simulink library "dspfdesign"  (Simulink 8.3)
settings: Solver=ode45  SolverMode=SingleTasking  StartTime=0.0  StopTime=10.0  RelTol=1e-3
undefined symbols (not defined in the file or in its folder): dfilt, fdesignblkfcn, gcbh
libraries: dsparch4 x4, dspmlti4 x1
settings Model: FPTRunName=Active  Creator=jschickl  LastModifiedBy=jibrahim  ExtModeAutoUpdateStatusClock=off

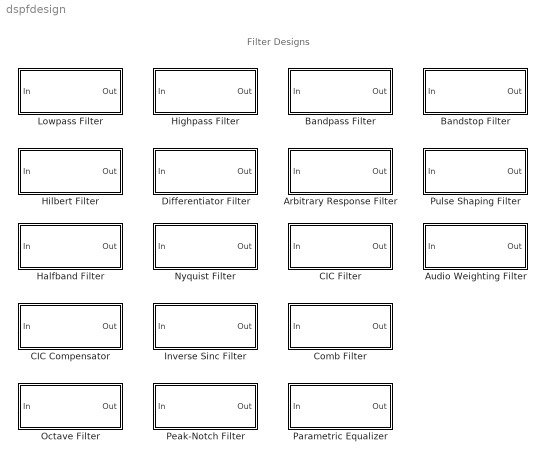
== system dspfdesign ==
  note: Filter Designs
  Arbitrary Response Filter : Subsystem  DialogController=fdesignblkfcn  DialogControllerArgs=DataTag1  InitFcn=fdesignblkfcn(gcbh, {'InitFcn'});  mask(Arbitrary Magnitude Filter){}
      mask help: Design an arbitrary magnitude filter
      settings: CopyFcn=fdesignblkfcn(gcbh, {'CopyFcn'});
      mask Help: helpview(mapfilelocation('dsp'), 'dsparbitrarymagnitudefilter');
      mask Display: disp('Arbitrary Response');
  Audio Weighting Filter : Subsystem  DialogController=fdesignblkfcn  DialogControllerArgs=DataTag3  InitFcn=fdesignblkfcn(gcbh, {'InitFcn'});  mask(Audio Weighting Filter){}
      mask help: Design an audio weighting filter
      settings: CopyFcn=fdesignblkfcn(gcbh, {'CopyFcn'});
      mask Help: helpview(mapfilelocation('dsp'), 'dspaudioweightingfilter');
      mask Display: disp('Audio Weighting')
  Bandpass Filter : Subsystem  DialogController=fdesignblkfcn  DialogControllerArgs=DataTag6  InitFcn=fdesignblkfcn(gcbh, {'InitFcn'});  mask(Bandpass Filter){}
      mask help: Design a bandpass filter
      settings: CopyFcn=fdesignblkfcn(gcbh, {'CopyFcn'});
      mask Help: helpview(mapfilelocation('dsp'), 'dspbandpassfilter');
      mask Display: disp('Bandpass');
  Bandstop Filter : Subsystem  DialogController=fdesignblkfcn  DialogControllerArgs=DataTag8  InitFcn=fdesignblkfcn(gcbh, {'InitFcn'});  mask(Bandstop Filter){}
      mask help: Design a bandstop filter
      settings: CopyFcn=fdesignblkfcn(gcbh, {'CopyFcn'});
      mask Help: helpview(mapfilelocation('dsp'), 'dspbandstopfilter');
      mask Display: disp('Bandstop');
  CIC Compensator : Subsystem  DialogController=fdesignblkfcn  DialogControllerArgs=DataTag10  InitFcn=fdesignblkfcn(gcbh, {'InitFcn'});  mask(CIC Compensator){}
      mask help: Design a CIC compensator
      settings: CopyFcn=fdesignblkfcn(gcbh, {'CopyFcn'});
      mask Help: helpview(mapfilelocation('dsp'), 'dspciccompensator');
      mask Display: disp('CIC Comp.')
  CIC Filter : Subsystem  DialogController=fdesignblkfcn  DialogControllerArgs=DataTag12  InitFcn=fdesignblkfcn(gcbh, {'InitFcn'});  mask(CIC Filter){}
      mask help: Design a CIC filter
      settings: CopyFcn=fdesignblkfcn(gcbh, {'CopyFcn'});
      mask Help: helpview(mapfilelocation('dsp'), 'dspcicfilter');
      mask Display: disp('CIC')
  Comb Filter : Subsystem  DialogController=fdesignblkfcn  DialogControllerArgs=DataTag15  InitFcn=fdesignblkfcn(gcbh, {'InitFcn'});  mask(Comb Filter){}
      mask help: Design a Comb Filter
      settings: CopyFcn=fdesignblkfcn(gcbh, {'CopyFcn'});
      mask Help: helpview(mapfilelocation('dsp'), 'dspcombfilter');
      mask Display: disp('Comb');
  Differentiator Filter : Subsystem  DialogController=fdesignblkfcn  DialogControllerArgs=DataTag17  InitFcn=fdesignblkfcn(gcbh, {'InitFcn'});  mask(Differentiator Filter){}
      mask help: Design a differentiator filter
      settings: CopyFcn=fdesignblkfcn(gcbh, {'CopyFcn'});
      mask Help: helpview(mapfilelocation('dsp'), 'dspdifferentiatorfilter');
      mask Display: disp('Differentiator');
  Halfband Filter : Subsystem  DialogController=fdesignblkfcn  DialogControllerArgs=DataTag19  InitFcn=fdesignblkfcn(gcbh, {'InitFcn'});  mask(Halfband Filter){}
      mask help: Design a halfband filter
      settings: CopyFcn=fdesignblkfcn(gcbh, {'CopyFcn'});
      mask Help: helpview(mapfilelocation('dsp'), 'dsphalfbandfilter');
      mask Display: disp('Halfband');
  Highpass Filter : Subsystem  DialogController=fdesignblkfcn  DialogControllerArgs=DataTag21  InitFcn=fdesignblkfcn(gcbh, {'InitFcn'});  mask(Highpass Filter){}
      mask help: Design a highpass filter
      settings: CopyFcn=fdesignblkfcn(gcbh, {'CopyFcn'});
      mask Help: helpview(mapfilelocation('dsp'), 'dsphighpassfilter');
      mask Display: disp('Highpass')
  Hilbert Filter : Subsystem  DialogController=fdesignblkfcn  DialogControllerArgs=DataTag23  InitFcn=fdesignblkfcn(gcbh, {'InitFcn'});  mask(Hilbert Filter){}
      mask help: Design a Hilbert filter
      settings: CopyFcn=fdesignblkfcn(gcbh, {'CopyFcn'});
      mask Help: helpview(mapfilelocation('dsp'), 'dsphilbertfilter');
      mask Display: disp('Hilbert')
  Inverse Sinc Filter : Subsystem  DialogController=fdesignblkfcn  DialogControllerArgs=DataTag25  InitFcn=fdesignblkfcn(gcbh, {'InitFcn'});  mask(Inverse Sinc Filter){}
      mask help: Design an inverse sinc filter
      settings: CopyFcn=fdesignblkfcn(gcbh, {'CopyFcn'});
      mask Help: helpview(mapfilelocation('dsp'), 'dspinversesincfilter');
      mask Display: disp('Inverse Sinc');
  Lowpass Filter : Subsystem  DialogController=fdesignblkfcn  DialogControllerArgs=DataTag27  InitFcn=fdesignblkfcn(gcbh, {'InitFcn'});  mask(Lowpass Filter){}
      mask help: Design a lowpass filter
      settings: CopyFcn=fdesignblkfcn(gcbh, {'CopyFcn'});
      mask Help: helpview(mapfilelocation('dsp'), 'dsplowpassfilter');
      mask Display: disp('Lowpass')
  Nyquist Filter : Subsystem  DialogController=fdesignblkfcn  DialogControllerArgs=DataTag29  InitFcn=fdesignblkfcn(gcbh, {'InitFcn'});  mask(Nyquist Filter){}
      mask help: Design a Nyquist filter
      settings: CopyFcn=fdesignblkfcn(gcbh, {'CopyFcn'});
      mask Help: helpview(mapfilelocation('dsp'), 'dspnyquistfilter');
      mask Display: disp('Nyquist');
  Octave Filter : Subsystem  DialogController=fdesignblkfcn  DialogControllerArgs=DataTag31  InitFcn=fdesignblkfcn(gcbh, {'InitFcn'});  mask(Octave Filter){}
      mask help: Design an octave filter
      settings: CopyFcn=fdesignblkfcn(gcbh, {'CopyFcn'});
      mask Help: helpview(mapfilelocation('dsp'), 'dspoctavefilter');
      mask Display: disp('Octave');
  Parametric Equalizer : Subsystem  DialogController=fdesignblkfcn  DialogControllerArgs=DataTag34  InitFcn=fdesignblkfcn(gcbh, {'InitFcn'});  mask(Parametric Equalizer){}
      mask help: Design a parametric equalizer
      settings: CopyFcn=fdesignblkfcn(gcbh, {'CopyFcn'});
      mask Help: helpview(mapfilelocation('dsp'), 'dspparametricequalizer');
      mask Display: disp('Param Eq');
  Peak-Notch Filter : Subsystem  DialogController=fdesignblkfcn  DialogControllerArgs=DataTag37  InitFcn=fdesignblkfcn(gcbh, {'InitFcn'});  mask(Peak/Notch Filter){}
      mask help: Design a peak/notch filter
      settings: CopyFcn=fdesignblkfcn(gcbh, {'CopyFcn'});
      mask Help: helpview(mapfilelocation('dsp'), 'dsppeaknotchfilter');
      mask Display: disp('Peak-Notch');
  Pulse Shaping Filter : Subsystem  DialogController=fdesignblkfcn  DialogControllerArgs=DataTag40  InitFcn=fdesignblkfcn(gcbh, {'InitFcn'});  mask(Pulse Shaping Filter){}
      mask help: Design a Pulse Shaping Filter
      settings: CopyFcn=fdesignblkfcn(gcbh, {'CopyFcn'});
      mask Help: helpview(mapfilelocation('dsp'), 'dsppulseshapingfilter');
      mask Display: disp('Pulse Shaping');

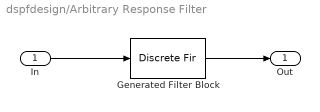
== system dspfdesign/Arbitrary Response Filter ==
  In : Inport
  Generated Filter Block : DiscreteFir  Tag=BlockMethodSubSystem  Coefficients=[-6.0602616490905374e-17 -0.030302449967817502 -2.7240579583698299e-18 -0.042316580413584839 1.9768060143351985e-17 -0.1094403863154082 6.5949666030061724e-17 0.28666822580143747 -9.0831528312516844e-17 0.093783802666672023 0.5 0.093783802666671731 1.4840405705753284e-16 0.28666822580143747 -1.1769252026794985e-16 -0.10944038631540809 3.1431295905226604e-17 -0.042316580413584826 -8.227645756848666e-17 -0.030302449967817453 1.2107664253565005e-16]  InputProcessing=Columns as channels (frame based)
  Out : Outport
  wires:
  In/1 -> Generated Filter Block/1
  Generated Filter Block/1 -> Out/1

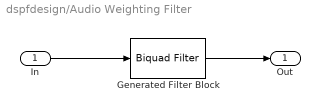
== system dspfdesign/Audio Weighting Filter ==
  In : Inport
  Generated Filter Block : dsparch4/Biquad Filter  Tag=BlockMethodSubSystem  IIRFiltStruct=Direct form II  CoeffSource=Specify via dialog  BiQuadCoeffs=[0.000322318592897719 0.000644637185795438 0.000322318592897719 1 -0.224558458059779 0.0126066252715464;1 -2 1 1 -1.89387049472307 0.895159769094661;1 -2 1 1 -1.99461445599302 0.994621707014084]  a0Flag=Warning  IC=0  ICnum=0  ICden=0  InputProcessing=Columns as channels (frame based)  denAccumFracLength=30  denProdOutputFracLength=30  secondMemoryFracLength=15  roundingMode=Floor  overflowMode=off  ScaleValues=[0.788048167211767;1;1;922.438644632257]  optimizeScaleValues=off  ScaleValueMode=Specify via input port (g)  scaleValueFracLength=14  FilterSource=Specify via dialog  dfiltObjectName=dfilt.df2tsos([1 0.3 0.4],[1 0.1 0.2])
  Out : Outport
  wires:
  Generated Filter Block/1 -> Out/1
  In/1 -> Generated Filter Block/1

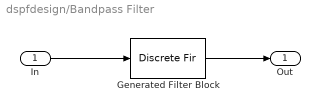
== system dspfdesign/Bandpass Filter ==
  In : Inport
  Generated Filter Block : DiscreteFir  Tag=BlockMethodSubSystem  Coefficients=[-0.0008992291487744296 0.0016414518747943749 0.0031352071842225397 -0.0040707550828814922 -0.0063731852227904111 0.0074874286806090491 0.0098354319566295711 -0.010189316513446216 -0.011302794465874122 0.0096929185841818435 0.0079428653987464216 -0.0031368247881221642 0.0028299878877943137 -0.011508674243001471 -0.022080136219461581 0.034245325424507672 0.048356661648905473 -0.062355369169884239 -0.077503478162593897 0.090687768153125653 0.10353171105844157 -0.11297860084229834 -0.12035866024978455 0.12379360801539134 0.12379360801539134 -0.12035866024978455 -0.11297860084229834 0.10353171105844157 0.090687768153125653 -0.077503478162593897 -0.062355369169884239 0.048356661648905473 0.034245325424507672 -0.022080136219461581 -0.011508674243001471 0.0028299878877943137 -0.0031368247881221642 0.0079428653987464216 0.0096929185841818435 -0.011302794465874122 -0.010189316513446216 0.0098354319566295711 0.0074874286806090491 -0.0063731852227904111 -0.0040707550828814922 0.0031352071842225397 0.0016414518747943749 -0.0008992291487744296]  InputProcessing=Columns as channels (frame based)
  Out : Outport
  wires:
  Generated Filter Block/1 -> Out/1
  In/1 -> Generated Filter Block/1

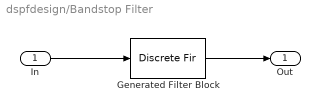
== system dspfdesign/Bandstop Filter ==
  In : Inport
  Generated Filter Block : DiscreteFir  Tag=BlockMethodSubSystem  Coefficients=[-0.00049984690227566171 9.5100318056220678e-05 -0.018778888889125381 0.00020561736622238936 0.0019605411941885044 0.00023848464356614288 0.011427768692370117 0.00024928020776728103 -0.026344143468356181 0.00022323473160311075 0.033802321854574921 0.00024455404571586617 -0.019823660150560137 0.00024377045334422507 -0.019896328302992174 0.00022786848806407702 0.082714162332194516 0.00025656261277749384 -0.15101859373266049 0.00022072984516862497 0.20526035643478094 0.0002476136866061962 0.77489283142488197 0.0002476136866061962 0.20526035643478094 0.00022072984516862497 -0.15101859373266049 0.00025656261277749384 0.082714162332194516 0.00022786848806407702 -0.019896328302992174 0.00024377045334422507 -0.019823660150560137 0.00024455404571586617 0.033802321854574921 0.00022323473160311075 -0.026344143468356181 0.00024928020776728103 0.011427768692370117 0.00023848464356614288 0.0019605411941885044 0.00020561736622238936 -0.018778888889125381 9.5100318056220678e-05 -0.00049984690227566171]  InputProcessing=Columns as channels (frame based)
  Out : Outport
  wires:
  In/1 -> Generated Filter Block/1
  Generated Filter Block/1 -> Out/1

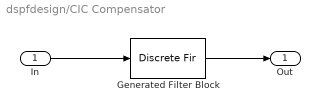
== system dspfdesign/CIC Compensator ==
  In : Inport
  Generated Filter Block : DiscreteFir  Tag=BlockMethodSubSystem  Coefficients=[-0.0050219629876821908 -0.013660028067670223 -0.013296841217015732 0.0011859158588442293 0.011467493725642241 -0.00013417577627168609 -0.013874989743002046 -0.0015600948868864728 0.0180127865455753 0.0042866842548780126 -0.023312910868604299 -0.0087360042158460029 0.030313491605369943 0.015598915258060758 -0.039779435104977612 -0.027013109649543846 0.054210638861692181 0.048428131419013934 -0.08074386512301486 -0.10321504031178634 0.15358183075835236 0.46749760644592786 0.46749760644592786 0.15358183075835236 -0.10321504031178634 -0.08074386512301486 0.048428131419013934 0.054210638861692181 -0.027013109649543846 -0.039779435104977612 0.015598915258060758 0.030313491605369943 -0.0087360042158460029 -0.023312910868604299 0.0042866842548780126 0.0180127865455753 -0.0015600948868864728 -0.013874989743002046 -0.00013417577627168609 0.011467493725642241 0.0011859158588442293 -0.013296841217015732 -0.013660028067670223 -0.0050219629876821908]  InputProcessing=Columns as channels (frame based)
  Out : Outport
  wires:
  In/1 -> Generated Filter Block/1
  Generated Filter Block/1 -> Out/1

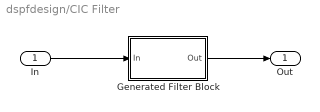
== system dspfdesign/CIC Filter ==
  In : Inport
  Generated Filter Block : Subsystem  Tag=BlockMethodSubSystem
  Out : Outport
  wires:
  Generated Filter Block/1(Out) -> Out/1
  In/1 -> Generated Filter Block/1(In)

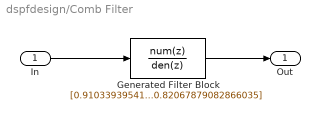
== system dspfdesign/Comb Filter ==
  In : Inport
  Generated Filter Block : DiscreteFilter  Tag=BlockMethodSubSystem  Numerator=[0.91033939541433018 0 0 0 0 0 0 0 0 0 -0.91033939541433018]  Denominator=[1 0 0 0 0 0 0 0 0 0 -0.82067879082866035]  InputProcessing=Columns as channels (frame based)
  Out : Outport
  wires:
  In/1 -> Generated Filter Block/1
  Generated Filter Block/1 -> Out/1

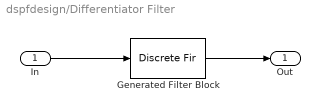
== system dspfdesign/Differentiator Filter ==
  In : Inport
  Generated Filter Block : DiscreteFir  Tag=BlockMethodSubSystem  Coefficients=[-0.0039403783503444709 0.0053805058704480841 -0.0026652365685344249 0.0025070872881500926 -0.0027292449144808066 0.0031396751895010648 -0.0037469771156754452 0.0046041330268851155 -0.0058435320681063689 0.007709493104211795 -0.010689468560152578 0.015879080885195844 -0.026138778807662393 0.051078874208799696 -0.14161732347277556 1.2733839756566323 -1.2733839756566323 0.14161732347277556 -0.051078874208799696 0.026138778807662393 -0.015879080885195844 0.010689468560152578 -0.007709493104211795 0.0058435320681063689 -0.0046041330268851155 0.0037469771156754452 -0.0031396751895010648 0.0027292449144808066 -0.0025070872881500926 0.0026652365685344249 -0.0053805058704480841 0.0039403783503444709]  InputProcessing=Columns as channels (frame based)
  Out : Outport
  wires:
  In/1 -> Generated Filter Block/1
  Generated Filter Block/1 -> Out/1

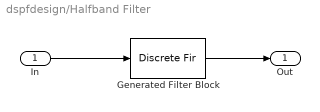
== system dspfdesign/Halfband Filter ==
  In : Inport
  Generated Filter Block : DiscreteFir  Tag=BlockMethodSubSystem  Coefficients=[-8.9481765259157725e-05 0 0.00013477350905337501 0 -0.0002322836857224922 0 0.00037237197523475751 0 -0.00056658311312798111 0 0.00082825383475131466 0 -0.0011725457806439315 0 0.0016168803439530585 0 -0.0021808856576991135 0 0.0028874400591769505 0 -0.0037630129230021257 0 0.0048394806436799498 0 -0.0061564154803690867 0 0.0077647763061666625 0 -0.009733715050901065 0 0.012161878543157797 0 -0.015198123798392082 0 0.019081615239417135 0 -0.024225970822374349 0 0.031415272990123339 0 -0.042336185081318312 0 0.061387315847790502 0 -0.10472460953008161 0 0.31784798756502125 0.5 0.31784798756502125 0 -0.10472460953008161 0 0.061387315847790502 0 -0.042336185081318312 0 0.031415272990123339 0 -0.024225970822374349 0 0.019081615239417135 0 -0.015198123798392082 0 0.012161878543157797 0 -0.009733715050901065 0 0.0077647763061666625 0 -0.0061564154803690867 0 0.0048394806436799498 0 -0.0037630129230021257 0 0.0028874400591769505 0 -0.0021808856576991135 0 0.0016168803439530585 0 -0.0011725457806439315 0 0.00082825383475131466 0 -0.00056658311312798111 0 0.00037237197523475751 0 -0.0002322836857224922 0 0.00013477350905337501 0 -8.9481765259157725e-05]  InputProcessing=Columns as channels (frame based)
  Out : Outport
  wires:
  In/1 -> Generated Filter Block/1
  Generated Filter Block/1 -> Out/1

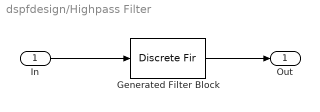
== system dspfdesign/Highpass Filter ==
  In : Inport
  Generated Filter Block : DiscreteFir  Tag=BlockMethodSubSystem  Coefficients=[-0.001713682665110306 0.0083143784480805769 -0.012717355233486931 0.0055609517902503753 0.0073397102425536197 -0.006531049050179258 -0.0076900499697794954 0.0090269831680985079 0.0088388618995090904 -0.012960741353766195 -0.010074958667252783 0.018520174010008873 0.011233354613588929 -0.026375248383613631 -0.012270782185765867 0.038180976692389727 0.013130425918293593 -0.058293359325192265 -0.013768295948648092 0.102813257992074 0.014167876773854067 -0.31720255241603534 0.48569804617051759 -0.31720255241603534 0.014167876773854067 0.102813257992074 -0.013768295948648092 -0.058293359325192265 0.013130425918293593 0.038180976692389727 -0.012270782185765867 -0.026375248383613631 0.011233354613588929 0.018520174010008873 -0.010074958667252783 -0.012960741353766195 0.0088388618995090904 0.0090269831680985079 -0.0076900499697794954 -0.006531049050179258 0.0073397102425536197 0.0055609517902503753 -0.012717355233486931 0.0083143784480805769 -0.001713682665110306]  InputProcessing=Columns as channels (frame based)
  Out : Outport
  wires:
  In/1 -> Generated Filter Block/1
  Generated Filter Block/1 -> Out/1

== system dspfdesign/Hilbert Filter ==
  In : Inport
  Generated Filter Block : DiscreteFir  Tag=BlockMethodSubSystem  Coefficients=[-0.026449858259791379 -0.00578355491829027 -0.016572261903348456 -0.0095390561131982743 -0.022461390535071568 -0.014999256435125952 -0.030323967074738556 -0.023012528163449009 -0.041429315821655127 -0.035762828939278346 -0.05911752381753177 -0.059034685410808696 -0.094459906652176406 -0.11739830204172252 -0.21797718993610349 -0.62869353747279177 0.62869353747279177 0.21797718993610349 0.11739830204172252 0.094459906652176406 0.059034685410808696 0.05911752381753177 0.035762828939278346 0.041429315821655127 0.023012528163449009 0.030323967074738556 0.014999256435125952 0.022461390535071568 0.0095390561131982743 0.016572261903348456 0.00578355491829027 0.026449858259791379]  InputProcessing=Columns as channels (frame based)
  Out : Outport
  wires:
  In/1 -> Generated Filter Block/1
  Generated Filter Block/1 -> Out/1

== system dspfdesign/Inverse Sinc Filter ==
  In : Inport
  Generated Filter Block : DiscreteFir  Tag=BlockMethodSubSystem  Coefficients=[-0.0026843274692852663 -0.002346162151096788 0.0073965993169508026 0.018442797618651186 0.012351106329410911 -0.0067934613704367722 -0.0093225132104399755 0.010137634289690594 0.014452636598032568 -0.01096659610710831 -0.020288876931548214 0.012277085521236011 0.029020142443779536 -0.013203596820367916 -0.042093940662690496 0.013627754834690312 0.064277570694568714 -0.012757715101713234 -0.11270171800644833 0.0051188971746040065 0.32344134739197722 0.50160314889955848 0.32344134739197722 0.0051188971746040065 -0.11270171800644833 -0.012757715101713234 0.064277570694568714 0.013627754834690312 -0.042093940662690496 -0.013203596820367916 0.029020142443779536 0.012277085521236011 -0.020288876931548214 -0.01096659610710831 0.014452636598032568 0.010137634289690594 -0.0093225132104399755 -0.0067934613704367722 0.012351106329410911 0.018442797618651186 0.0073965993169508026 -0.002346162151096788 -0.0026843274692852663]  InputProcessing=Columns as channels (frame based)
  Out : Outport
  wires:
  In/1 -> Generated Filter Block/1
  Generated Filter Block/1 -> Out/1

== system dspfdesign/Lowpass Filter ==
  In : Inport
  Generated Filter Block : DiscreteFir  Tag=BlockMethodSubSystem  Coefficients=[-0.0024228738523269142 -0.002083244982079274 0.0067703446401187091 0.016731945423489058 0.011117076081077608 -0.0062311454141445394 -0.008401617186026911 0.0092567976151380175 0.012982883808855752 -0.010121234703278968 -0.018273518733782485 0.011431962071777957 0.02617588858040763 -0.012489027835322923 -0.037996623145463579 0.013388945199366963 0.058155465814729891 -0.014048043515808939 -0.10272466857882172 0.014462275771238358 0.31716649721769491 0.48538764678732504 0.31716649721769491 0.014462275771238358 -0.10272466857882172 -0.014048043515808939 0.058155465814729891 0.013388945199366963 -0.037996623145463579 -0.012489027835322923 0.02617588858040763 0.011431962071777957 -0.018273518733782485 -0.010121234703278968 0.012982883808855752 0.0092567976151380175 -0.008401617186026911 -0.0062311454141445394 0.011117076081077608 0.016731945423489058 0.0067703446401187091 -0.002083244982079274 -0.0024228738523269142]  InputProcessing=Columns as channels (frame based)
  Out : Outport
  wires:
  Generated Filter Block/1 -> Out/1
  In/1 -> Generated Filter Block/1

== system dspfdesign/Nyquist Filter ==
  In : Inport
  Generated Filter Block : DiscreteFir  Tag=BlockMethodSubSystem  Coefficients=[-1.5162272612995586e-05 0 4.1706564279713027e-05 0 -8.6397453235949307e-05 0 0.00015611233941239259 0 -0.00025915216340561289 0 0.00040534096772710702 0 -0.00060612208112690072 0 0.00087466461351889491 0 -0.0012260032157642615 0 0.0016772472887656247 0 -0.0022479153417375975 0 0.002960480176087802 0 -0.0038412587047380814 0 0.0049218611113159959 0 -0.0062415564318662039 0 0.0078511744671022864 0 -0.0098196745838436145 0 0.012245562776669343 0 -0.015277650505299337 0 0.019155163922055268 0 -0.024291754943524414 0 0.031471599148898237 0 -0.042381607242685339 0 0.061420660829271646 0 -0.10474499179295332 0 0.31785484611193615 0.5 0.31785484611193615 0 -0.10474499179295332 0 0.061420660829271646 0 -0.042381607242685339 0 0.031471599148898237 0 -0.024291754943524414 0 0.019155163922055268 0 -0.015277650505299337 0 0.012245562776669343 0 -0.0098196745838436145 0 0.0078511744671022864 0 -0.0062415564318662039 0 0.0049218611113159959 0 -0.0038412587047380814 0 0.002960480176087802 0 -0.0022479153417375975 0 0.0016772472887656247 0 -0.0012260032157642615 0 0.00087466461351889491 0 -0.00060612208112690072 0 0.00040534096772710702 0 -0.00025915216340561289 0 0.00015611233941239259 0 -8.6397453235949307e-05 0 4.1706564279713027e-05 0 -1.5162272612995586e-05]  InputProcessing=Columns as channels (frame based)
  Out : Outport
  wires:
  Generated Filter Block/1 -> Out/1
  In/1 -> Generated Filter Block/1

== system dspfdesign/Octave Filter ==
  In : Inport
  Generated Filter Block : dsparch4/Biquad Filter  Tag=BlockMethodSubSystem  IIRFiltStruct=Direct form II  CoeffSource=Specify via dialog  BiQuadCoeffs=[0.115971860617354 0 -0.115971860617354 1 -1.95883566965961 0.967994525760731;0.0548911505711939 0 -0.0548911505711939 1 -1.91157093401714 0.942106946582538;2 0 -2 1 -1.89540803000166 0.911775131877275]  a0Flag=Warning  IC=0  ICnum=0  ICden=0  InputProcessing=Columns as channels (frame based)  denAccumFracLength=30  denProdOutputFracLength=30  secondMemoryFracLength=15  roundingMode=Floor  overflowMode=off  ScaleValues=[0.00304051963098346;1;1;2.31504954634773]  optimizeScaleValues=off  ScaleValueMode=Specify via input port (g)  scaleValueFracLength=14  FilterSource=Specify via dialog  dfiltObjectName=dfilt.df2tsos([1 0.3 0.4],[1 0.1 0.2])
  Out : Outport
  wires:
  In/1 -> Generated Filter Block/1
  Generated Filter Block/1 -> Out/1

== system dspfdesign/Parametric Equalizer ==
  In : Inport
  Generated Filter Block : dsparch4/Biquad Filter  Tag=BlockMethodSubSystem  IIRFiltStruct=Direct form II  CoeffSource=Specify via dialog  BiQuadCoeffs=[0.848020960436601 0.659110935021998 0.38962445572443 1 0.55108714605605 0.621190092613526;1.60063898438456 -1.24407144027101 0.735415894414984 1 -0.551087146056049 0.621190092613524]  a0Flag=Warning  IC=0  ICnum=0  ICden=0  InputProcessing=Columns as channels (frame based)  denAccumFracLength=30  denProdOutputFracLength=30  secondMemoryFracLength=15  roundingMode=Floor  overflowMode=off  ScaleValues=[0.35490589484659;1;1]  optimizeScaleValues=off  ScaleValueMode=Specify via input port (g)  scaleValueFracLength=14  FilterSource=Specify via dialog  dfiltObjectName=dfilt.df2tsos([1 0.3 0.4],[1 0.1 0.2])
  Out : Outport
  wires:
  In/1 -> Generated Filter Block/1
  Generated Filter Block/1 -> Out/1

== system dspfdesign/Peak-Notch Filter ==
  In : Inport
  Generated Filter Block : dsparch4/Biquad Filter  Tag=BlockMethodSubSystem  IIRFiltStruct=Direct form II  CoeffSource=Specify via dialog  BiQuadCoeffs=[0.38547134611574 -0.77094269223148 0.38547134611574 1 0.476387796295706 0.738730881654112;0.307522030597872 -4.58243541688184e-09 -0.307522026015436 1 -0.476387796295706 0.73873088165411;0.608203917574429 1.2164078442118 0.608203926637374 1 0 0.509525449494429]  a0Flag=Warning  IC=0  ICnum=0  ICden=0  InputProcessing=Columns as channels (frame based)  denAccumFracLength=30  denProdOutputFracLength=30  secondMemoryFracLength=15  roundingMode=Floor  overflowMode=off  ScaleValues=[0.251035664112808;1;1;1]  optimizeScaleValues=off  ScaleValueMode=Specify via input port (g)  scaleValueFracLength=14  FilterSource=Specify via dialog  dfiltObjectName=dfilt.df2tsos([1 0.3 0.4],[1 0.1 0.2])
  Out : Outport
  wires:
  In/1 -> Generated Filter Block/1
  Generated Filter Block/1 -> Out/1

== system dspfdesign/Pulse Shaping Filter ==
  In : Inport
  Generated Filter Block : DiscreteFir  Tag=BlockMethodSubSystem  Coefficients=[-6.2159943453401388e-35 -2.6765867803437917e-05 -0.00010512162870520087 -0.00021655697685248282 -0.000324789435843112 -0.00038511600235498363 -0.00035845025523960843 -0.00022605072067271852 3.2484765270994796e-19 0.00027497269129193083 0.00053064358359394695 0.00069450089893466284 0.00071453675885484592 0.00058237001544539791 0.00034644156669813477 0.00010844327316896579 1.1188789821612247e-34 0.00014220821937304821 0.0005965993733009448 0.0013207595841003069 0.0021436102765645384 0.002773203749015552 0.0028437053582342255 0.0019989975494783549 -1.6242382635497397e-18 -0.0031661141311613732 -0.0072015914916321319 -0.011464607147029125 -0.015005271935951766 -0.016676959533209128 -0.015312717248057542 -0.0099406333738218545 3.8270212473354788e-18 0.014484922916140437 0.032812965531551885 0.053622839114472479 0.075026359679758847 0.094843568216331872 0.11090450897113481 0.12136770836118578 0.125 0.12136770836118578 0.11090450897113481 0.094843568216331872 0.075026359679758847 0.053622839114472479 0.032812965531551885 0.014484922916140437 3.8270212473354788e-18 -0.0099406333738218545 -0.015312717248057542 -0.016676959533209128 -0.015005271935951766 -0.011464607147029125 -0.0072015914916321319 -0.0031661141311613732 -1.6242382635497397e-18 0.0019989975494783549 0.0028437053582342255 0.002773203749015552 0.0021436102765645384 0.0013207595841003069 0.0005965993733009448 0.00014220821937304821 1.1188789821612247e-34 0.00010844327316896579 0.00034644156669813477 0.00058237001544539791 0.00071453675885484592 0.00069450089893466284 0.00053064358359394695 0.00027497269129193083 3.2484765270994796e-19 -0.00022605072067271852 -0.00035845025523960843 -0.00038511600235498363 -0.000324789435843112 -0.00021655697685248282 -0.00010512162870520087 -2.6765867803437917e-05 -6.2159943453401388e-35]  InputProcessing=Columns as channels (frame based)
  Out : Outport
  wires:
  Generated Filter Block/1 -> Out/1
  In/1 -> Generated Filter Block/1

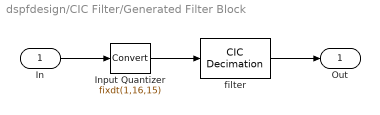
== system dspfdesign/CIC Filter/Generated Filter Block ==
  In : Inport
  Input Quantizer : DataTypeConversion  OutDataTypeStr=fixdt(1,16,15)  RndMeth=Round  SaturateOnIntegerOverflow=on
  filter : dspmlti4/CIC Decimation  filtFrom=Dialog  filtobj=Hm_decim  ftype=Decimator  R=2  M=1  N=2  filterInternals=Full precision  BPS=[18 18 18 18]  FLPS=[15 15 15 15]  outputWordLength=18  outputFracLength=15  launchFVT=off  framing=Maintain input frame rate  RateOptions=Enforce single-rate processing
  Out : Outport
  wires:
  filter/1 -> Out/1
  Input Quantizer/1 -> filter/1
  In/1 -> Input Quantizer/1
